simulink model "double_pend_cart_sfun"  (R2020a)
settings: Solver=VariableStepAuto  StartTime=0.0  StopTime=10.0  RelTol=1e-3
settings Model: Creator=Tomo  LastModifiedBy=Tomo

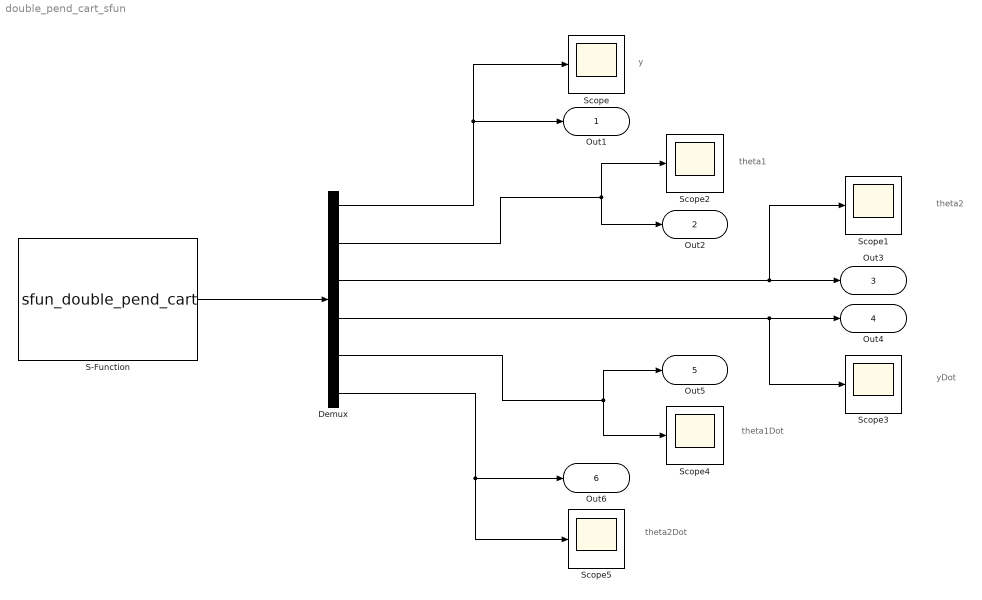
== system double_pend_cart_sfun ==
  note: y
  note: theta1
  note: yDot
  note: theta2
  note: theta1Dot
  note: theta2Dot
  Demux : Demux  Outputs=6
  S-Function : S-Function  FunctionName=sfun_double_pend_cart  SFunctionDeploymentMode=off  EnableBusSupport=off
  Scope{,1..5} (6 alike) : Scope
  Out1 : Outport
  Out2 : Outport  Port=2
  Out3 : Outport  Port=3
  Out4 : Outport  Port=4
  Out5 : Outport  Port=5
  Out6 : Outport  Port=6
  wires:
  Demux/1 -> Out1/1, Scope/1
  Demux/2 -> Out2/1, Scope2/1
  Demux/3 -> Scope1/1, Out3/1
  Demux/4 -> Scope3/1, Out4/1
  Demux/5 -> Out5/1, Scope4/1
  Demux/6 -> Scope5/1, Out6/1
  S-Function/1 -> Demux/1
